simulink model "slave_task"  (Simulink 7.1)
libraries: mathlib x4, inoutlib x1
settings Model: Creator=jsobota  LastModifiedBy=jsobota  ExtModeTrigMode=oneshot  ExtModeArmWhenConnect=off

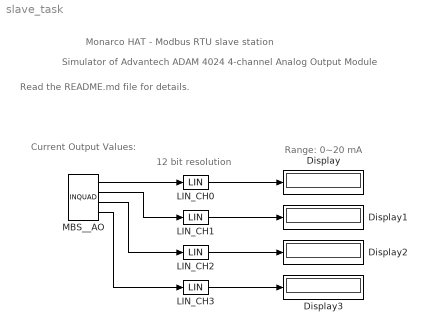
== system slave_task ==
  note: Range: 0~20 mA
  note: 12 bit resolution
  note: Current Output Values:
  note: Read the README.md file for details.
  note: Simulator of Advantech ADAM 4024 4-channel Analog Output Module
  note: Monarco HAT - Modbus RTU slave station
  Display{,1..3} (4 alike) : Display
      settings: Format=short
  LIN_CH{0..3} (4 alike) : mathlib/LIN  u1=0  y1=0  u2=4095  y2=20
  MBS__AO : inoutlib/INQUAD
  wires:
  LIN_CH0/1 -> Display/1
  LIN_CH1/1 -> Display1/1
  LIN_CH2/1 -> Display2/1
  LIN_CH3/1 -> Display3/1
  MBS__AO/1 -> LIN_CH0/1
  MBS__AO/2 -> LIN_CH1/1
  MBS__AO/3 -> LIN_CH2/1
  MBS__AO/4 -> LIN_CH3/1
